simulink model "VDCHyd2020a"  (R2020a)
settings: Solver=daessc  StartTime=0.0  StopTime=simulationEndTime  FixedStep=0.001  RelTol=1e-2
values from neighbouring files (symbols this model uses):
  Bc1_V = [0;0;0;0;0;0]    [initializeSimulationGP.m]
  filtDV = init2ndOrderLowPassFilter(35*2*pi,1,controller.dT)    [initializeLowPassFilters.m]
  filtEnc = init2ndOrderLowPassFilter(35*2*pi,1,controller.dT)    [initializeLowPassFilters.m]
undefined symbols (not defined in the file or in its folder): aux, B11_r_B11Tc1, B11_V, B11_Vr, B11Ftot_r, B12_r_B12Tc2, B12_Rot_Tc2, B12_U_Tc2, B12_V, B12_Vr, B12Ftot_r, B31_r_B31B41, B31_V, B31_Vr, B31FTot_r, B32_r_B32B42, B32_Rot_B42, B32_U_B42, B32_V, B32_Vr, B32FTot_r, B41_r_B41Tc1, B41_V, B41_Vr, B41FTot_r, B42_r_B42Tc2, B42_Rot_Tc2, B42_U_Tc2, B42_V, B42_Vr, B42FTot_r, B52_r_B52P32, B52_Rot_P32, B52_U_P32, B52_V, B52_Vr, B52Ftot_r, Bc1_r_Bc1B11, Bc1_r_Bc1B31, Bc1_Vr, Bc1FTot_r, Bc2_r_Bc2B12, Bc2_r_Bc2B32, Bc2_Rot_B12, Bc2_Rot_B32, Bc2_U_B12, Bc2_U_B32, Bc2_V, Bc2_Vr, Bc2Tot_r, controller, cyl1, cyl2, cylT2, D22_V, D22_Vr, D22Fr, DiscIntNeverNeededParam, dq1, dq11 ... (+125)
libraries: sm_lib x34, nesl_utility x15, simulink x11, dspinverses x1
(part 5 of 12)

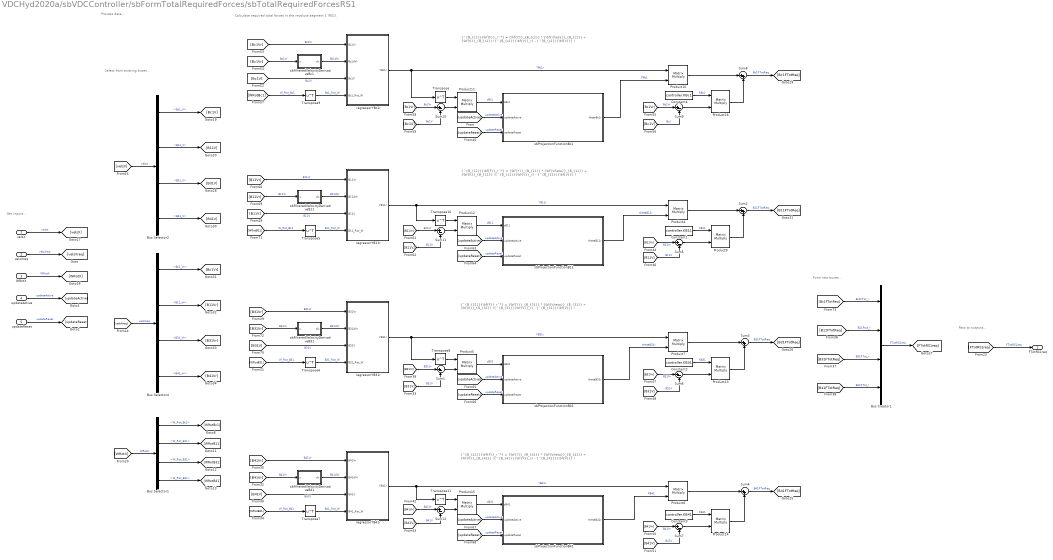
== system VDCHyd2020a/sbVDCController/sbFormTotalRequiredForces/sbTotalRequiredForcesRS1 ==
  note: {^{B_{c1}}{\bf{F}}_r^*} = {\bf{Y}}_{B_{c1}} * {\bf{\theta}}_{B_{c1}} + {\bf{K}}_{B_{c1}} ({^{B_{c1}}{\bf{V}}_r} - {^{B_{c1}}{\bf{V}}} )
  note: Select from existing buses...
  note: Process data...
  note: Get inputs...
  note: Pass to outputs...
  note: Calculate required total forces in the revolute segment 1 (RS1).
  note: Form new buses...
  note: {^{B_{11}}{\bf{F}}_r^*} = {\bf{Y}}_{B_{11}} * {\bf{\theta}}_{B_{11}} + {\bf{K}}_{B_{11}} ({^{B_{11}}{\bf{V}}_r} - {^{B_{11}}{\bf{V}}} )
  note: {^{B_{31}}{\bf{F}}_r^*} = {\bf{Y}}_{B_{31}} * {\bf{\theta}}_{B_{31}} + {\bf{K}}_{B_{31}} ({^{B_{31}}{\bf{V}}_r} - {^{B_{31}}{\bf{V}}} )
  note: {^{B_{41}}{\bf{F}}_r^*} = {\bf{Y}}_{B_{41}} * {\bf{\theta}}_{B_{41}} + {\bf{K}}_{B_{41}} ({^{B_{41}}{\bf{V}}_r} - {^{B_{41}}{\bf{V}}} )
  velsX : Inport
  velsXreq : Inport  Port=2
  WRotX : Inport  Port=3
  updateActive : Inport  Port=4
  updateReset : Inport  Port=5
  Bus Creator1 : BusCreator  Inputs=Bc1FTot_r,B11Ftot_r,B31FTot_r,B41FTot_r
  Bus Selector1 : BusSelector  OutputSignals=WRotXRS1.W_Rot_Bc1,WRotXRS1.W_Rot_B11,WRotXRS1.W_Rot_B31,WRotXRS1.W_Rot_B41
  Bus Selector2 : BusSelector  OutputSignals=velsRS1.Bc1_V,velsRS1.B11_V,velsRS1.B31_V,velsRS1.B41_V
  Bus Selector4 : BusSelector  OutputSignals=velsRS1req.Bc1_Vr,velsRS1req.B11_Vr,velsRS1req.B31_Vr,velsRS1req.B41_Vr
  Constant1 : Constant  Value=controller.KB11
  Constant2 : Constant  Value=controller.KB31
  Constant3 : Constant  Value=controller.KB41
  Constant4 : Constant  Value=controller.KBc1
  Product{4..7,9..16} (12 alike) : Product  Multiplication=Matrix(*)
  Sum{1,5..7,9..12} (8 alike) : Sum  Inputs=|+-
  Sum{2..4,8} (4 alike) : Sum  Inputs=|++
  Transpose{,5..11} (8 alike) : Math  Operator=transpose  SaturateOnIntegerOverflow=on
  regressorYB11r : MATLAB Function  TreatAsAtomicUnit=on
  regressorYB31r : MATLAB Function  TreatAsAtomicUnit=on
  regressorYB41r : MATLAB Function  TreatAsAtomicUnit=on
  regressorYBc1r : MATLAB Function  TreatAsAtomicUnit=on
  sbFilteredVelocityDerivativeB11 : Subsystem
  sbFilteredVelocityDerivativeB31 : Subsystem
  sbFilteredVelocityDerivativeB41 : Subsystem
  sbFilteredVelocityDerivativeBc1 : Subsystem
  sbProjectionFunctionB11 : Subsystem
  sbProjectionFunctionB31 : Subsystem
  sbProjectionFunctionB41 : Subsystem
  sbProjectionFunctionBc1 : Subsystem
  FTotRS1req : Outport
  wires:
  [FTotRS1req] -> FTotRS1req/1  "FTotRS1req"
  velsX/1 -> [velsX]  "velsX"
  [WRotX] -> Bus Selector1/1  "WRotX"
  WRotX/1 -> [WRotX]  "WRotX"
  Bus Selector1/4 -> [WRotB41]  "<W_Rot_B41>"
  Bus Selector1/2 -> [WRotB11]  "<W_Rot_B11>"
  Bus Selector1/1 -> [WRotBc1]  "<W_Rot_Bc1>"
  Bus Selector1/3 -> [WRotB31]  "<W_Rot_B31>"
  regressorYB31r/1(YB31r) -> Transpose8/1, Product7/1  "YB31r"
  [updateReset] -> sbProjectionFunctionB31/3(updateReset)  "updateReset"
  sbFilteredVelocityDerivativeB31/1(du) -> regressorYB31r/2(B31dVr)  "B31dVr"
  [B11V] -> Sum11/2  "B11V"
  [B41V] -> Sum7/2  "B41V"
  [velsX] -> Bus Selector2/1  "velsX"
  [B31V] -> Sum6/2  "B31V"
  Bus Selector4/4 -> [B41Vr]  "<B41_Vr>"
  sbFilteredVelocityDerivativeB41/1(du) -> regressorYB41r/2(B41dVr)  "B41dVr"
  Sum10/1 -> Product11/2
  sbProjectionFunctionB31/1(thetaB31r) -> Product7/2  "thetaB31r"
  Bus Creator1/1 -> [FTotRS1req]  "FTotRS1req"
  Bus Selector4/2 -> [B11Vr]  "<B11_Vr>"
  Bus Selector4/3 -> [B31Vr]  "<B31_Vr>"
  Sum5/1 -> Product9/2
  Sum8/1 -> [Bc1FTotReq]  "Bc1FTotReq"
  [Bc1FTotReq] -> Bus Creator1/1  "Bc1FTot_r"
  [WRotB31] -> Transpose6/1  "W_Rot_B31"
  [B41FTotReq] -> Bus Creator1/4  "B41FTot_r"
  [updateReset] -> sbProjectionFunctionB41/3(updateReset)  "updateReset"
  Bus Selector2/1 -> [Bc1V]  "<Bc1_V>"
  [B31FTotReq] -> Bus Creator1/3  "B31FTot_r"
  Product12/1 -> sbProjectionFunctionB11/1(sB11)  "sB11"
  [WRotBc1] -> Transpose9/1  "W_Rot_Bc1"
  Transpose5/1 -> regressorYB11r/4(B11_Rot_W)  "B11_Rot_W"
  [Bc1Vr] -> Sum9/1  "Bc1Vr"
  [B41Vr] -> regressorYB41r/1(B41Vr)  "B41Vr"
  [B41V] -> Sum12/2  "B41V"
  Transpose/1 -> Product11/1
  [WRotB11] -> Transpose5/1  "W_Rot_B11"
  Bus Selector2/2 -> [B11V]  "<B11_V>"
  [updateReset] -> sbProjectionFunctionBc1/3(updateReset)  "updateReset"
  Bus Selector2/4 -> [B41V]  "<B41_V>"
  [B11Vr] -> regressorYB11r/1(B11Vr)  "B11Vr"
  [Bc1V] -> Sum10/2  "Bc1V"
  Transpose10/1 -> Product12/1
  Sum11/1 -> Product12/2
  [Bc1V] -> regressorYBc1r/3(Bc1V)  "Bc1V"
  regressorYBc1r/1(YBc1r) -> Product10/1, Transpose/1  "YBc1r"
  Product10/1 -> Sum8/1
  Product11/1 -> sbProjectionFunctionBc1/1(sBc1)  "sBc1"
  Transpose8/1 -> Product5/1
  Bus Selector4/1 -> [Bc1Vr]  "<Bc1_Vr>"
  [B11Vr] -> Sum11/1  "B11Vr"
  Product9/1 -> Sum2/2
  Product7/1 -> Sum3/1
  [B31Vr] -> Sum1/1  "B31Vr"
  Sum6/1 -> Product13/2
  [B41Vr] -> Sum7/1  "B41Vr"
  Sum12/1 -> Product15/2
  [updateActive] -> sbProjectionFunctionBc1/2(updateActive)  "updateActive"
  regressorYB11r/1(YB11r) -> Transpose10/1, Product4/1  "YB11r"
  regressorYB41r/1(YB41r) -> Product6/1, Transpose11/1  "YB41r"
  [B41Vr] -> Sum12/1  "B41Vr"
  sbProjectionFunctionBc1/1(thetaBc1r) -> Product10/2  "PBc1"
  Transpose11/1 -> Product15/1
  [WRotB41] -> Transpose7/1  "W_Rot_B41"
  sbFilteredVelocityDerivativeB11/1(du) -> regressorYB11r/2(B11dVr)  "B11dVr"
  [Bc1Vr] -> sbFilteredVelocityDerivativeBc1/1(u)  "Bc1Vr"
  [B41V] -> regressorYB41r/3(B41V)  "B41V"
  Sum7/1 -> Product14/2
  Product15/1 -> sbProjectionFunctionB41/1(sB41)  "sB41"
  [B11Vr] -> Sum5/1  "B11Vr"
  [B31Vr] -> regressorYB31r/1(B31Vr)  "B31Vr"
  [Bc1Vr] -> Sum10/1  "Bc1Vr"
  Constant1/1 -> Product9/1  "KB11"
  [B11V] -> regressorYB11r/3(B11V)  "B11V"
  Transpose7/1 -> regressorYB41r/4(B41_Rot_W)  "B41_Rot_W"
  Transpose9/1 -> regressorYBc1r/4(Bc1_Rot_W)  "Bc1_Rot_W"
  Sum1/1 -> Product5/2
  [B11FTotReq] -> Bus Creator1/2  "B11Ftot_r"
  [B31Vr] -> sbFilteredVelocityDerivativeB31/1(u)  "B31Vr"
  Product6/1 -> Sum4/1
  [B11V] -> Sum5/2  "B11V"
  Product14/1 -> Sum4/2
  [updateActive] -> sbProjectionFunctionB41/2(updateActive)  "updateActive"
  [updateReset] -> sbProjectionFunctionB11/3(updateReset)  "updateReset"
  [velsXreq] -> Bus Selector4/1  "velsXreq"
  Bus Selector2/3 -> [B31V]  "<B31_V>"
  [Bc1Vr] -> regressorYBc1r/1(Bc1Vr)  "Bc1Vr"
  [B31V] -> regressorYB31r/3(B31V)  "B31V"
  sbProjectionFunctionB11/1(thetaB11r) -> Product4/2  "thetaB11r"
  [B41Vr] -> sbFilteredVelocityDerivativeB41/1(u)  "B41Vr"
  Sum9/1 -> Product16/2
  sbFilteredVelocityDerivativeBc1/1(du) -> regressorYBc1r/2(Bc1dVr)  "Bc1dVr"
  Constant4/1 -> Product16/1  "KBc1"
  Constant3/1 -> Product14/1  "KB41"
  Product5/1 -> sbProjectionFunctionB31/1(sB31)  "sB31"
  Sum4/1 -> [B41FTotReq]  "B41FTotReq"
  [B31Vr] -> Sum6/1  "B31Vr"
  [Bc1V] -> Sum9/2  "Bc1"
  Transpose6/1 -> regressorYB31r/4(B31_Rot_W)  "B31_Rot_W"
  [updateActive] -> sbProjectionFunctionB11/2(updateActive)  "updateActive"
  Product16/1 -> Sum8/2
  [B31V] -> Sum1/2  "B31V"
  Product13/1 -> Sum3/2
  Product4/1 -> Sum2/1
  [B11Vr] -> sbFilteredVelocityDerivativeB11/1(u)  "B11Vr"
  Constant2/1 -> Product13/1  "KB31"
  Sum2/1 -> [B11FTotReq]  "B11FTotReq"
  sbProjectionFunctionB41/1(thetaB41r) -> Product6/2  "PB41"
  Sum3/1 -> [B31FTotReq]  "B31FTotReq"
  [updateActive] -> sbProjectionFunctionB31/2(updateActive)  "updateActive"
  velsXreq/1 -> [velsXreq]  "velsXreq"
  updateActive/1 -> [updateActive]  "updateActive"
  updateReset/1 -> [updateReset]  "updateReset"

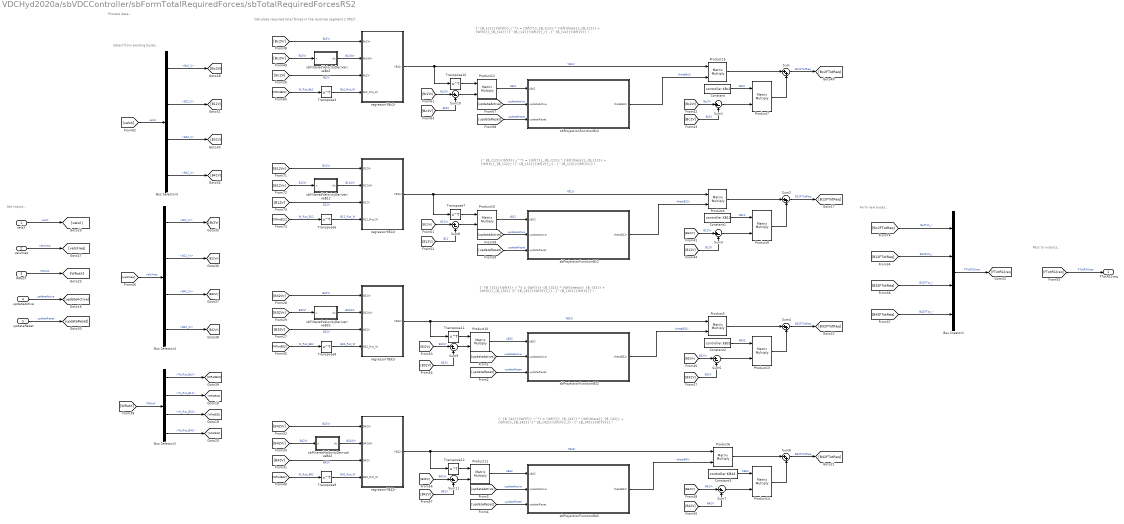
== system VDCHyd2020a/sbVDCController/sbFormTotalRequiredForces/sbTotalRequiredForcesRS2 ==
  note: Form new buses...
  note: Calculate required total forces in the revolute segment 2 (RS2).
  note: Select from existing buses...
  note: Process data...
  note: Pass to outputs...
  note: Get inputs...
  note: {^{B_{c2}}{\bf{F}}_r^*} = {\bf{Y}}_{B_{c2}} * {\bf{\theta}}_{B_{c2}} + {\bf{K}}_{B_{c2}} ({^{B_{c2}}{\bf{V}}_r} - {^{B_{c2}}{\bf{V}}} )
  note: {^{B_{12}}{\bf{F}}_r^*} = {\bf{Y}}_{B_{12}} * {\bf{\theta}}_{B_{12}} + {\bf{K}}_{B_{12}} ({^{B_{12}}{\bf{V}}_r} - {^{B_{12}}{\bf{V}}} )
  note: {^{B_{32}}{\bf{F}}_r^*} = {\bf{Y}}_{B_{32}} * {\bf{\theta}}_{B_{32}} + {\bf{K}}_{B_{32}} ({^{B_{32}}{\bf{V}}_r} - {^{B_{32}}{\bf{V}}} )
  note: {^{B_{42}}{\bf{F}}_r^*} = {\bf{Y}}_{B_{42}} * {\bf{\theta}}_{B_{42}} + {\bf{K}}_{B_{42}} ({^{B_{42}}{\bf{V}}_r} - {^{B_{42}}{\bf{V}}} )
  velsX : Inport
  velsXreq : Inport  Port=2
  WRotX : Inport  Port=3
  updateActive : Inport  Port=4
  updateReset : Inport  Port=5
  Bus Creator1 : BusCreator  Inputs=Bc2Tot_r,B12Ftot_r,B32FTot_r,B42FTot_r
  Bus Selector2 : BusSelector  OutputSignals=WRotXRS1.W_Rot_Bc2,WRotXRS2.W_Rot_B12,WRotXRS2.W_Rot_B32,WRotXRS2.W_Rot_B42
  Bus Selector3 : BusSelector  OutputSignals=velsRS2.Bc2_V,velsRS2.B12_V,velsRS2.B32_V,velsRS2.B42_V
  Bus Selector4 : BusSelector  OutputSignals=velsRS1req.Bc2_Vr,velsRS2req.B12_Vr,velsRS2req.B42_Vr,velsRS2req.B32_Vr
  Constant : Constant  Value=controller.KBc2
  Constant1 : Constant  Value=controller.KB12
  Constant2 : Constant  Value=controller.KB32
  Constant3 : Constant  Value=controller.KB42
  Product{4..7,9..16} (12 alike) : Product  Multiplication=Matrix(*)
  Sum{,2,4,6} (4 alike) : Sum  Inputs=|++
  Sum{1,3,5,7..11} (8 alike) : Sum  Inputs=|+-
  Transpose{3,6..12} (8 alike) : Math  Operator=transpose  SaturateOnIntegerOverflow=on
  regressorYB12r : MATLAB Function  TreatAsAtomicUnit=on
  regressorYB32r : MATLAB Function  TreatAsAtomicUnit=on
  regressorYB42r : MATLAB Function  TreatAsAtomicUnit=on
  regressorYBc2r : MATLAB Function  TreatAsAtomicUnit=on
  sbFilteredVelocityDerivativeB12 : Subsystem
  sbFilteredVelocityDerivativeB32 : Subsystem
  sbFilteredVelocityDerivativeB42 : Subsystem
  sbFilteredVelocityDerivativeBc2 : Subsystem
  sbProjectionFunctionB12 : Subsystem
  sbProjectionFunctionB32 : Subsystem
  sbProjectionFunctionB42 : Subsystem
  sbProjectionFunctionBc2 : Subsystem
  FTotRS2req : Outport
  wires:
  Bus Selector3/1 -> [Bc2V]  "<Bc2_V>"
  Bus Selector2/1 -> [WRotBc2]  "<W_Rot_Bc2>"
  [B42Vr] -> Sum7/1  "B42Vr"
  Product7/1 -> Sum/2
  Bus Creator1/1 -> [FTotRS2req]  "FTotRS2req"
  [B12V] -> regressorYB12r/3(B12V)  "B12V"
  [Bc2V] -> regressorYBc2r/3(Bc2V)  "Bc2V"
  [B32FTotReq] -> Bus Creator1/3  "B32FTot_r"
  [WRotX] -> Bus Selector2/1  "WRotX"
  Transpose10/1 -> Product12/1
  sbProjectionFunctionB12/1(thetaB12r) -> Product4/2  "thetaB12r"
  [Bc2Vr] -> Sum1/1  "Bc2Vr"
  [FTotRS2req] -> FTotRS2req/1  "FTotRS2req"
  [B42FTotReq] -> Bus Creator1/4  "B42FTot_r"
  [Bc2FTotReq] -> Bus Creator1/1  "Bc2Tot_r"
  [B32V] -> Sum9/2  "B32V"
  Sum4/1 -> [B32FTotReq]  "B32FTotReq"
  Bus Selector2/2 -> [WRotB12]  "<W_Rot_B12>"
  [B12Vr] -> Sum3/1  "B12Vr"
  Bus Selector2/4 -> [WRotB42]  "<W_Rot_B42>"
  Transpose6/1 -> regressorYB12r/4(B12_Rot_W)  "B12_Rot_W"
  Sum7/1 -> Product14/2
  [B32Vr] -> sbFilteredVelocityDerivativeB32/1(u)  "B32Vr"
  [WRotB32] -> Transpose8/1  "W_Rot_B32"
  sbFilteredVelocityDerivativeB32/1(du) -> regressorYB32r/2(B32dVr)  "B32dVr"
  [B32Vr] -> regressorYB32r/1(B32Vr)  "B32Vr"
  Product4/1 -> Sum2/1
  [B12Vr] -> Sum8/1  "B12Vr"
  Sum/1 -> [Bc2FTotReq]  "Bc2FTotReq"
  [B42Vr] -> sbFilteredVelocityDerivativeB42/1(u)  "B42Vr"
  [B42Vr] -> regressorYB42r/1(B42Vr)  "B42Vr"
  Constant2/1 -> Product13/1  "KB32"
  Transpose9/1 -> regressorYB42r/4(B42_Rot_W)  "B42_Rot_W"
  [B42V] -> regressorYB42r/3(B42V)  "B42V"
  Constant1/1 -> Product9/1  "KB12"
  [updateReset] -> sbProjectionFunctionB12/3(updateReset)  "updateReset"
  sbProjectionFunctionB32/1(thetaB32r) -> Product5/2  "thetaB32r"
  [updateActive] -> sbProjectionFunctionBc2/2(updateActive)  "updateActive"
  Sum5/1 -> Product13/2
  Sum3/1 -> Product9/2
  Product13/1 -> Sum4/2
  Product11/1 -> sbProjectionFunctionB42/1(sB42)  "sB42"
  Product14/1 -> Sum6/2
  Sum6/1 -> [B42FTotReq]  "B42FTotReq"
  Sum1/1 -> Product7/2
  [B32Vr] -> Sum5/1  "B32Vr"
  Product9/1 -> Sum2/2
  [updateReset] -> sbProjectionFunctionBc2/3(updateReset)  "updateReset"
  Constant3/1 -> Product14/1  "KB42"
  Sum10/1 -> Product12/2
  [Bc2Vr] -> Sum10/1  "Bc2Vr"
  Transpose7/1 -> Product16/1
  [B32Vr] -> Sum9/1  "B32Vr"
  regressorYB32r/1(YB32r) -> Transpose11/1, Product5/1  "YB32r"
  regressorYBc2r/1(YBc2r) -> Product15/1, Transpose10/1  "YBc2r"
  Product16/1 -> sbProjectionFunctionB12/1(sB12)  "sB12"
  [Bc2V] -> Sum10/2  "Bc2V"
  Product5/1 -> Sum4/1
  Transpose11/1 -> Product10/1
  updateReset/1 -> [updateReset]  "updateReset"
  Product12/1 -> sbProjectionFunctionBc2/1(sBc2)  "sBc2"
  [updateActive] -> sbProjectionFunctionB12/2(updateActive)  "updateActive"
  Product10/1 -> sbProjectionFunctionB32/1(sB32)  "sB32"
  [Bc2V] -> Sum1/2  "Bc2V"
  Bus Selector4/4 -> [B42Vr]  "<B32_Vr>"
  [B32V] -> Sum5/2  "B32V"
  sbProjectionFunctionB42/1(thetaB42r) -> Product6/2  "thetaB42r"
  sbProjectionFunctionBc2/1(thetaBc2r) -> Product15/2  "thetaBc2r"
  regressorYB12r/1(YB12r) -> Product4/1, Transpose7/1  "YB12r"
  [velsX] -> Bus Selector3/1  "velsX"
  [WRotB42] -> Transpose9/1  "W_Rot_B42"
  Transpose12/1 -> Product11/1
  regressorYB42r/1(YB42r) -> Product6/1, Transpose12/1  "YB42r"
  Bus Selector3/4 -> [B42V]  "<B42_V>"
  WRotX/1 -> [WRotX]  "WRotX"
  [B12Vr] -> sbFilteredVelocityDerivativeB12/1(u)  "B12Vr"
  Transpose8/1 -> regressorYB32r/4(B32_Rot_W)  "B32_Rot_W"
  Sum9/1 -> Product10/2
  [B42V] -> Sum11/2  "B42V"
  Bus Selector2/3 -> [WRotB32]  "<W_Rot_B32>"
  updateActive/1 -> [updateActive]  "updateActive"
  [WRotBc2] -> Transpose3/1  "W_Rot_Bc2"
  [velsXreq] -> Bus Selector4/1  "velsXreq"
  [B12V] -> Sum8/2  "B12"
  sbFilteredVelocityDerivativeBc2/1(du) -> regressorYBc2r/2(Bc2dVr)  "Bc2dVr"
  Sum8/1 -> Product16/2
  Sum11/1 -> Product11/2
  Sum2/1 -> [B12FTotReq]  "B12FTotReq"
  Bus Selector4/1 -> [Bc2Vr]  "<Bc2_Vr>"
  Constant/1 -> Product7/1  "KBc2"
  [B12V] -> Sum3/2  "B12V"
  [B12Vr] -> regressorYB12r/1(B12Vr)  "B12Vr"
  [Bc2Vr] -> regressorYBc2r/1(Bc2Vr)  "Bc2Vr"
  [B32V] -> regressorYB32r/3(B32V)  "B32V"
  [B42V] -> Sum7/2  "B42V"
  Product6/1 -> Sum6/1
  [WRotB12] -> Transpose6/1  "W_Rot_B12"
  sbFilteredVelocityDerivativeB42/1(du) -> regressorYB42r/2(B42dVr)  "B42dVr"
  sbFilteredVelocityDerivativeB12/1(du) -> regressorYB12r/2(B12dVr)  "B12dVr"
  [B42Vr] -> Sum11/1  "B42Vr"
  Bus Selector3/2 -> [B12V]  "<B12_V>"
  Bus Selector3/3 -> [B32V]  "<B32_V>"
  [Bc2Vr] -> sbFilteredVelocityDerivativeBc2/1(u)  "Bc2Vr"
  Bus Selector4/3 -> [B32Vr]  "<B42_Vr>"
  velsX/1 -> [velsX]  "velsX"
  Transpose3/1 -> regressorYBc2r/4(Bc2_Rot_W)  "Bc2_Rot_W"
  Product15/1 -> Sum/1
  Bus Selector4/2 -> [B12Vr]  "<B12_Vr>"
  velsXreq/1 -> [velsXreq]  "velsXreq"
  [B12FTotReq] -> Bus Creator1/2  "B12Ftot_r"
  [updateReset] -> sbProjectionFunctionB32/3(updateReset)  "updateReset"
  [updateActive] -> sbProjectionFunctionB32/2(updateActive)  "updateActive"
  [updateActive] -> sbProjectionFunctionB42/2(updateActive)  "updateActive"
  [updateReset] -> sbProjectionFunctionB42/3(updateReset)  "updateReset"

== system VDCHyd2020a/sbVDCController/sbFormingControlActions/sbDiscreteDerivativefp1r ==
  fp1r : Inport
  Add : Sum  Inputs=-+
  Gain6 : Gain  Gain=1/(2*controller.dT)
  Integer Delay : Delay  InitialConditionSource=Input port  InitialCondition=0  SampleTime=controller.dT
      settings: InputPortMap=u0,p4
  dfp1r : Outport  PortDimensions=1
  wires:
  Add/1 -> Gain6/1
  fp1r/1 -> Integer Delay/1, Integer Delay/2, Add/2
  Integer Delay/1 -> Add/1
  Gain6/1 -> dfp1r/1

== system VDCHyd2020a/sbVDCController/sbFormingControlActions/sbDiscreteDerivativefp2r ==
  fp2r : Inport
  Add : Sum  Inputs=-+
  Gain6 : Gain  Gain=1/(2*controller.dT)
  Integer Delay : Delay  InitialConditionSource=Input port  InitialCondition=0  SampleTime=controller.dT
      settings: InputPortMap=u0,p4
  dfp2r : Outport  PortDimensions=1
  wires:
  Add/1 -> Gain6/1
  fp2r/1 -> Integer Delay/1, Integer Delay/2, Add/2
  Integer Delay/1 -> Add/1
  Gain6/1 -> dfp2r/1

== system VDCHyd2020a/sbVDCController/sbFormingControlActions/sbDiscreteDerivativefpt2r ==
  fpt2r : Inport
  Add : Sum  Inputs=-+
  Gain6 : Gain  Gain=1/(2*controller.dT)
  Integer Delay : Delay  InitialConditionSource=Input port  InitialCondition=0  SampleTime=controller.dT
      settings: InputPortMap=u0,p4
  dfpt2r : Outport  PortDimensions=1
  wires:
  Gain6/1 -> dfpt2r/1
  Integer Delay/1 -> Add/1
  fpt2r/1 -> Add/2, Integer Delay/2, Integer Delay/1
  Add/1 -> Gain6/1

== system VDCHyd2020a/sbVDCController/sbFormingControlActions/sbFrictionRegressorPS2 ==
  note: (40) in Zhu, Piedboeuf (2005)
  note: (4) in Zhu, Piedboeuf (2005)
  note: (71) and (72) in Zhu, Piedboeuf (2005)
  dxt2 : Inport
  fpt2 : Inport  Port=2
  frictionRegressorFunctionPS2 : MATLAB Function  TreatAsAtomicUnit=on
  sbAverageDeformationOfBristlesPS2 : Subsystem
  sbFrictionSwitchingFunctionPS2 : Subsystem
  Yft2 : Outport
  wires:
  dxt2/1 -> [dxt2]  "dxt2"
  [dxt2] -> sbAverageDeformationOfBristlesPS2/1(dxt2)  "dxt2"
  sbAverageDeformationOfBristlesPS2/1(zt2) -> [zt2]  "zt2"
  [dxt2] -> sbFrictionSwitchingFunctionPS2/1(dxt2)  "dxt2"
  sbFrictionSwitchingFunctionPS2/1(LPS2) -> [LPS2]  "LPS2"
  [dxt2] -> frictionRegressorFunctionPS2/1(v)  "dxt2"
  [zt2] -> frictionRegressorFunctionPS2/2(z)  "zt2"
  [LPS2] -> frictionRegressorFunctionPS2/3(L)  "LPS2"
  fpt2/1 -> [fpt2]  "fpt2"
  [fpt2] -> frictionRegressorFunctionPS2/4(Fd)  "fpt2"
  frictionRegressorFunctionPS2/1(Yf) -> [Yft2]  "Yft2"
  [Yft2] -> Yft2/1  "Yft2"

== system VDCHyd2020a/sbVDCController/sbFormingControlActions/sbFrictionRegressorRS1 ==
  note: (40) in Zhu, Piedboeuf (2005)
  note: (4) in Zhu, Piedboeuf (2005)
  note: (71) and (72) in Zhu, Piedboeuf (2005)
  dx1 : Inport
  fp1 : Inport  Port=2
  frictionRegressorFunctionRS1 : MATLAB Function  TreatAsAtomicUnit=on
  sbAverageDeformationOfBristlesRS2 : Subsystem
  sbFrictionSwitchingFunctionRS2 : Subsystem
  Yf1 : Outport
  wires:
  dx1/1 -> [dx1]  "dx1"
  [dx1] -> sbAverageDeformationOfBristlesRS2/1(dx1)  "dx1"
  sbAverageDeformationOfBristlesRS2/1(z1) -> [z1]  "z1"
  [dx1] -> sbFrictionSwitchingFunctionRS2/1(dx1)  "dx1"
  sbFrictionSwitchingFunctionRS2/1(LRS1) -> [LRS1]  "LRS1"
  [dx1] -> frictionRegressorFunctionRS1/1(v)  "dx1"
  [z1] -> frictionRegressorFunctionRS1/2(z)  "z1"
  [LRS1] -> frictionRegressorFunctionRS1/3(L)  "LRS1"
  fp1/1 -> [fp1]  "fp1"
  [fp1] -> frictionRegressorFunctionRS1/4(Fd)  "fp1"
  frictionRegressorFunctionRS1/1(Yf) -> [Yf1]  "Yf1"
  [Yf1] -> Yf1/1  "Yf1"

== system VDCHyd2020a/sbVDCController/sbFormingControlActions/sbFrictionRegressorRS2 ==
  note: (40) in Zhu, Piedboeuf (2005)
  note: (4) in Zhu, Piedboeuf (2005)
  note: (71) and (72) in Zhu, Piedboeuf (2005)
  dx2 : Inport
  fp2 : Inport  Port=2
  frictionRegressorFunctionRS2 : MATLAB Function  TreatAsAtomicUnit=on
  sbAverageDeformationOfBristlesRS2 : Subsystem
  sbFrictionSwitchingFunctionRS2 : Subsystem
  Yf2 : Outport
  wires:
  dx2/1 -> [dx2]  "dx2"
  [dx2] -> sbAverageDeformationOfBristlesRS2/1(dx2)  "dx2"
  sbAverageDeformationOfBristlesRS2/1(z2) -> [z2]  "z2"
  [dx2] -> sbFrictionSwitchingFunctionRS2/1(dx2)  "dx2"
  sbFrictionSwitchingFunctionRS2/1(LRS2) -> [LRS2]  "LRS2"
  [dx2] -> frictionRegressorFunctionRS2/1(v)  "dx2"
  [z2] -> frictionRegressorFunctionRS2/2(z)  "z2"
  [LRS2] -> frictionRegressorFunctionRS2/3(L)  "LRS2"
  fp2/1 -> [fp2]  "fp2"
  [fp2] -> frictionRegressorFunctionRS2/4(Fd)  "fp2"
  frictionRegressorFunctionRS2/1(Yf) -> [Yf2]  "Yf2"
  [Yf2] -> Yf2/1  "Yf2"

== system VDCHyd2020a/sbVDCController/sbFormingControlActions/sbLowPassFilter2 ==
  dfp2r : Inport
  Delay : Delay  InitialConditionSource=Input port  SampleTime=filtDF.dT
      settings: InputPortMap=u0,p4
  Delay1 : Delay  DelayLength=1  InitialConditionSource=Input port  SampleTime=filtDF.dT
      settings: InputPortMap=u0,p4
  Delay2 : Delay  DelayLength=0  InitialConditionSource=Input port  SampleTime=filtDF.dT
      settings: InputPortMap=u0,p4
  Delay3 : Delay  InitialConditionSource=Input port  SampleTime=filtDF.dT
      settings: InputPortMap=u0,p4
  Delay4 : Delay  DelayLength=1  InitialConditionSource=Input port  SampleTime=filtDF.dT
      settings: InputPortMap=u0,p4
  Gain : Gain  Gain=filtDF.a0
  Gain1 : Gain  Gain=filtDF.b1
  Gain2 : Gain  Gain=filtDF.b2
  Gain3 : Gain  Gain=filtDF.b0
  Gain4 : Gain  Gain=filtDF.a1
  Sum : Sum  Inputs=|--+++
  dfp2rFilt : Outport
  wires:
  Delay2/1 -> Gain2/1
  Delay3/1 -> Gain3/1
  Gain1/1 -> Sum/4
  Delay/1 -> Gain/1
  Gain2/1 -> Sum/3
  Gain3/1 -> Sum/5
  Sum/1 -> dfp2rFilt/1, Delay4/1, Delay/1  "df2pFilt"
  Gain4/1 -> Sum/1
  Delay1/1 -> Gain1/1
  Delay4/1 -> Gain4/1
  Gain/1 -> Sum/2
  dfp2r/1 -> Delay4/2, Delay/2, Delay2/1, Delay2/2, Delay1/1, Delay3/2, Delay3/1, Delay1/2  "df2p"

== system VDCHyd2020a/sbVDCController/sbFormingControlActions/sbLowPassFilterdfp1r ==
  dfp1r : Inport
  Delay : Delay  InitialConditionSource=Input port  SampleTime=filtDF.dT
      settings: InputPortMap=u0,p4
  Delay1 : Delay  DelayLength=1  InitialConditionSource=Input port  SampleTime=filtDF.dT
      settings: InputPortMap=u0,p4
  Delay2 : Delay  DelayLength=0  InitialConditionSource=Input port  SampleTime=filtDF.dT
      settings: InputPortMap=u0,p4
  Delay3 : Delay  InitialConditionSource=Input port  SampleTime=filtDF.dT
      settings: InputPortMap=u0,p4
  Delay4 : Delay  DelayLength=1  InitialConditionSource=Input port  SampleTime=filtDF.dT
      settings: InputPortMap=u0,p4
  Gain : Gain  Gain=filtDF.a0
  Gain1 : Gain  Gain=filtDF.b1
  Gain2 : Gain  Gain=filtDF.b2
  Gain3 : Gain  Gain=filtDF.b0
  Gain4 : Gain  Gain=filtDF.a1
  Sum : Sum  Inputs=|--+++
  dfp1rFilt : Outport
  wires:
  dfp1r/1 -> Delay1/2, Delay3/1, Delay3/2, Delay1/1, Delay2/2, Delay2/1, Delay/2, Delay4/2  "df1p"
  Gain/1 -> Sum/2
  Delay4/1 -> Gain4/1
  Delay1/1 -> Gain1/1
  Gain4/1 -> Sum/1
  Sum/1 -> Delay/1, Delay4/1, dfp1rFilt/1  "df1pFilt"
  Gain3/1 -> Sum/5
  Gain2/1 -> Sum/3
  Delay/1 -> Gain/1
  Gain1/1 -> Sum/4
  Delay3/1 -> Gain3/1
  Delay2/1 -> Gain2/1

== system VDCHyd2020a/sbVDCController/sbFormingControlActions/sbLowPassFilterdfpt2r ==
  dfpt2r : Inport
  Delay : Delay  InitialConditionSource=Input port  SampleTime=filtDF.dT
      settings: InputPortMap=u0,p4
  Delay1 : Delay  DelayLength=1  InitialConditionSource=Input port  SampleTime=filtDF.dT
      settings: InputPortMap=u0,p4
  Delay2 : Delay  DelayLength=0  InitialConditionSource=Input port  SampleTime=filtDF.dT
      settings: InputPortMap=u0,p4
  Delay3 : Delay  InitialConditionSource=Input port  SampleTime=filtDF.dT
      settings: InputPortMap=u0,p4
  Delay4 : Delay  DelayLength=1  InitialConditionSource=Input port  SampleTime=filtDF.dT
      settings: InputPortMap=u0,p4
  Gain : Gain  Gain=filtDF.a0
  Gain1 : Gain  Gain=filtDF.b1
  Gain2 : Gain  Gain=filtDF.b2
  Gain3 : Gain  Gain=filtDF.b0
  Gain4 : Gain  Gain=filtDF.a1
  Sum : Sum  Inputs=|--+++
  dfpt2rFilt : Outport
  wires:
  dfpt2r/1 -> Delay1/2, Delay3/1, Delay3/2, Delay1/1, Delay2/2, Delay2/1, Delay/2, Delay4/2  "dft2p"
  Gain/1 -> Sum/2
  Delay4/1 -> Gain4/1
  Delay1/1 -> Gain1/1
  Gain4/1 -> Sum/1
  Sum/1 -> Delay/1, Delay4/1, dfpt2rFilt/1  "dft2pFilt"
  Gain3/1 -> Sum/5
  Gain2/1 -> Sum/3
  Delay/1 -> Gain/1
  Gain1/1 -> Sum/4
  Delay3/1 -> Gain3/1
  Delay2/1 -> Gain2/1

== system VDCHyd2020a/sbVDCController/sbFormingControlActions/sbProjectionFunctiond1 ==
  sd1 : Inport  PortDimensions=4
  updateActive : Inport  Port=2
  updateReset : Inport  Port=3
  Constant1 : Constant  Value=update.thetad1Nominal
  Switch1 : Switch  Criteria=u2 > Threshold
  discreteIntegratorPd1 : DiscreteIntegrator  IntegratorMethod=Integration: Trapezoidal  gainval=update.rhod1  ExternalReset=level  InitialConditionSource=external  InitialCondition=update.thetad1Nominal  SampleTime=controller.dT  LimitOutput=on  UpperSaturationLimit=update.thetad1UpperBound  LowerSaturationLimit=update.thetad1LowerBound  ICPrevOutput=DiscIntNeverNeededParam  ICPrevScaledInput=DiscIntNeverNeededParam
  thetad1 : Outport
  wires:
  sd1/1 -> discreteIntegratorPd1/1  "sd1"
  updateReset/1 -> discreteIntegratorPd1/2  "updateReset"
  discreteIntegratorPd1/1 -> Switch1/1  "thetad1Updated"
  Switch1/1 -> thetad1/1  "thetad1"
  updateActive/1 -> Switch1/2  "updateActive"
  Constant1/1 -> discreteIntegratorPd1/3, Switch1/3  "thetad1Nominal"

== system VDCHyd2020a/sbVDCController/sbFormingControlActions/sbProjectionFunctiond2 ==
  sd2 : Inport  PortDimensions=4
  updateActive : Inport  Port=2
  updateReset : Inport  Port=3
  Constant1 : Constant  Value=update.thetad2Nominal
  Switch1 : Switch  Criteria=u2 > Threshold
  discreteIntegratorPd2 : DiscreteIntegrator  IntegratorMethod=Integration: Trapezoidal  gainval=update.rhod2  ExternalReset=level  InitialConditionSource=external  InitialCondition=update.thetad2Nominal  SampleTime=controller.dT  LimitOutput=on  UpperSaturationLimit=update.thetad2UpperBound  LowerSaturationLimit=update.thetad2LowerBound  ICPrevOutput=DiscIntNeverNeededParam  ICPrevScaledInput=DiscIntNeverNeededParam
  thetad2 : Outport
  wires:
  Constant1/1 -> Switch1/3, discreteIntegratorPd2/3  "thetad2Nominal"
  updateActive/1 -> Switch1/2  "updateActive"
  Switch1/1 -> thetad2/1  "thetad2"
  discreteIntegratorPd2/1 -> Switch1/1  "thetad2Updated"
  updateReset/1 -> discreteIntegratorPd2/2  "updateReset"
  sd2/1 -> discreteIntegratorPd2/1  "sd2"

== system VDCHyd2020a/sbVDCController/sbFormingControlActions/sbProjectionFunctiondt2 ==
  sdt2 : Inport  PortDimensions=4
  updateActive : Inport  Port=2
  updateReset : Inport  Port=3
  Constant1 : Constant  Value=update.thetadT2Nominal
  Discrete-Time Integrator : DiscreteIntegrator  IntegratorMethod=Integration: Trapezoidal  gainval=update.rhodT2  ExternalReset=level  InitialConditionSource=external  InitialCondition=update.thetadT2Nominal  SampleTime=controller.dT  LimitOutput=on  UpperSaturationLimit=update.thetadT2UpperBound  LowerSaturationLimit=update.thetadT2LowerBound  ICPrevOutput=DiscIntNeverNeededParam  ICPrevScaledInput=DiscIntNeverNeededParam
  Switch1 : Switch  Criteria=u2 > Threshold
  thetadT2 : Outport
  wires:
  sdt2/1 -> Discrete-Time Integrator/1  "sdt2"
  updateReset/1 -> Discrete-Time Integrator/2  "updateReset"
  Discrete-Time Integrator/1 -> Switch1/1  "thetadT2Updated"
  Switch1/1 -> thetadT2/1  "thetadT2"
  updateActive/1 -> Switch1/2  "updateActive"
  Constant1/1 -> Switch1/3, Discrete-Time Integrator/3  "thetadT2Nominal"

== system VDCHyd2020a/sbVDCController/sbFormingControlActions/sbProjectionFunctionfRS1 ==
  sf1 : Inport
  updateActive : Inport  Port=2
  updateReset : Inport  Port=3
  Constant1 : Constant  Value=update.thetaf1Nominal
  Switch1 : Switch  Criteria=u2 > Threshold
  discreteIntegratorPf1 : DiscreteIntegrator  IntegratorMethod=Integration: Trapezoidal  gainval=update.rhof1  ExternalReset=level  InitialConditionSource=external  InitialCondition=update.thetaf1Nominal  SampleTime=controller.dT  LimitOutput=on  UpperSaturationLimit=update.thetaf1UpperBound  LowerSaturationLimit=update.thetaf1LowerBound  ICPrevOutput=DiscIntNeverNeededParam  ICPrevScaledInput=DiscIntNeverNeededParam
  thetaf1 : Outport
  wires:
  sf1/1 -> discreteIntegratorPf1/1  "sf1"
  updateReset/1 -> discreteIntegratorPf1/2  "updateReset"
  discreteIntegratorPf1/1 -> Switch1/1  "thetaf1Updated"
  Switch1/1 -> thetaf1/1  "thetaf1"
  updateActive/1 -> Switch1/2  "updateActive"
  Constant1/1 -> discreteIntegratorPf1/3, Switch1/3  "thetaf1Nominal"

== system VDCHyd2020a/sbVDCController/sbFormingControlActions/sbProjectionFunctionfRS2 ==
  sf2 : Inport
  updateActive : Inport  Port=2
  updateReset : Inport  Port=3
  Constant1 : Constant  Value=update.thetaf2Nominal
  Switch1 : Switch  Criteria=u2 > Threshold
  discreteIntegratorPf2 : DiscreteIntegrator  IntegratorMethod=Integration: Trapezoidal  gainval=update.rhof2  ExternalReset=level  InitialConditionSource=external  InitialCondition=update.thetaf2Nominal  SampleTime=controller.dT  LimitOutput=on  UpperSaturationLimit=update.thetaf2UpperBound  LowerSaturationLimit=update.thetaf2LowerBound  ICPrevOutput=DiscIntNeverNeededParam  ICPrevScaledInput=DiscIntNeverNeededParam
  thetaf2 : Outport
  wires:
  Constant1/1 -> Switch1/3, discreteIntegratorPf2/3  "thetaf2Nominal"
  updateActive/1 -> Switch1/2  "updateActive"
  Switch1/1 -> thetaf2/1  "thetaf2"
  discreteIntegratorPf2/1 -> Switch1/1  "thetaf2Updated"
  updateReset/1 -> discreteIntegratorPf2/2  "updateReset"
  sf2/1 -> discreteIntegratorPf2/1  "sf2"

== system VDCHyd2020a/sbVDCController/sbFormingControlActions/sbProjectionFunctionfRS3 ==
  sfT2 : Inport
  updateActive : Inport  Port=2
  updateReset : Inport  Port=3
  Constant1 : Constant  Value=update.thetafT2Nominal
  Switch1 : Switch  Criteria=u2 > Threshold
  discreteIntegratorPfT2 : DiscreteIntegrator  IntegratorMethod=Integration: Trapezoidal  gainval=update.rhofT2  ExternalReset=level  InitialConditionSource=external  InitialCondition=update.thetafT2Nominal  SampleTime=controller.dT  LimitOutput=on  UpperSaturationLimit=update.thetafT2UpperBound  LowerSaturationLimit=update.thetafT2LowerBound  ICPrevOutput=DiscIntNeverNeededParam  ICPrevScaledInput=DiscIntNeverNeededParam
  thetafT2 : Outport
  wires:
  sfT2/1 -> discreteIntegratorPfT2/1  "sfT2"
  updateReset/1 -> discreteIntegratorPfT2/2  "updateReset"
  discreteIntegratorPfT2/1 -> Switch1/1  "thetaf2Updated"
  Switch1/1 -> thetafT2/1  "thetafT2"
  updateActive/1 -> Switch1/2  "updateActive"
  Constant1/1 -> discreteIntegratorPfT2/3, Switch1/3  "thetafT2Nominal"

== system VDCHyd2020a/sbVDCController/sbFormingControlActions/sbProjectionFunctionv1 ==
  sv1 : Inport  PortDimensions=4
  updateActive : Inport  Port=2
  updateReset : Inport  Port=3
  Constant1 : Constant  Value=update.thetav1Nominal
  Switch1 : Switch  Criteria=u2 > Threshold
  Unit Delay : UnitDelay  InitialCondition=update.thetav1Nominal  SampleTime=controller.dT  HasFrameUpgradeWarning=on
  discreteIntegratorPv1 : DiscreteIntegrator  IntegratorMethod=Integration: Trapezoidal  gainval=update.rhov1  ExternalReset=level  InitialConditionSource=external  InitialCondition=update.thetav1Nominal  SampleTime=controller.dT  LimitOutput=on  UpperSaturationLimit=update.thetav1UpperBound  LowerSaturationLimit=update.thetav1LowerBound  ICPrevOutput=DiscIntNeverNeededParam  ICPrevScaledInput=DiscIntNeverNeededParam
  thetav1 : Outport
  wires:
  Constant1/1 -> discreteIntegratorPv1/3, Switch1/3  "thetav1Nominal"
  updateActive/1 -> Switch1/2  "updateActive"
  Switch1/1 -> thetav1/1  "thetav1"
  discreteIntegratorPv1/1 -> Unit Delay/1
  updateReset/1 -> discreteIntegratorPv1/2  "updateReset"
  sv1/1 -> discreteIntegratorPv1/1  "sv1"
  Unit Delay/1 -> Switch1/1  "thetav1Update"

== system VDCHyd2020a/sbVDCController/sbFormingControlActions/sbProjectionFunctionv2 ==
  sv2 : Inport  PortDimensions=4
  updateActive : Inport  Port=2
  updateReset : Inport  Port=3
  Constant1 : Constant  Value=update.thetav2Nominal
  Discrete-Time Integrator : DiscreteIntegrator  IntegratorMethod=Integration: Trapezoidal  gainval=update.rhov2  ExternalReset=level  InitialConditionSource=external  InitialCondition=update.thetav2Nominal  SampleTime=controller.dT  LimitOutput=on  UpperSaturationLimit=update.thetav2UpperBound  LowerSaturationLimit=update.thetav2LowerBound  ICPrevOutput=DiscIntNeverNeededParam  ICPrevScaledInput=DiscIntNeverNeededParam
  Switch1 : Switch  Criteria=u2 > Threshold
  Unit Delay : UnitDelay  InitialCondition=update.thetav2Nominal  SampleTime=controller.dT  HasFrameUpgradeWarning=on
  thetav2 : Outport
  wires:
  Constant1/1 -> Switch1/3, Discrete-Time Integrator/3  "thetav2Nominal"
  updateActive/1 -> Switch1/2  "updateActive"
  Switch1/1 -> thetav2/1  "thetav2"
  Discrete-Time Integrator/1 -> Unit Delay/1
  updateReset/1 -> Discrete-Time Integrator/2  "updateReset"
  sv2/1 -> Discrete-Time Integrator/1  "sv2"
  Unit Delay/1 -> Switch1/1  "thetav2Updated"

== system VDCHyd2020a/sbVDCController/sbFormingControlActions/sbProjectionFunctionvt2 ==
  svt2 : Inport  PortDimensions=4
  updateActive : Inport  Port=2
  updateReset : Inport  Port=3
  Constant1 : Constant  Value=update.thetavT2Nominal
  Discrete-Time Integrator : DiscreteIntegrator  IntegratorMethod=Integration: Trapezoidal  gainval=update.rhovT2  ExternalReset=level  InitialConditionSource=external  InitialCondition=update.thetavT2Nominal  SampleTime=controller.dT  LimitOutput=on  UpperSaturationLimit=update.thetavT2UpperBound  LowerSaturationLimit=update.thetavT2LowerBound  ICPrevOutput=DiscIntNeverNeededParam  ICPrevScaledInput=DiscIntNeverNeededParam
  Switch1 : Switch  Criteria=u2 > Threshold
  Unit Delay : UnitDelay  InitialCondition=update.thetavT2Nominal  SampleTime=controller.dT  HasFrameUpgradeWarning=on
  thetavt2 : Outport
  wires:
  svt2/1 -> Discrete-Time Integrator/1
  Switch1/1 -> thetavt2/1  "thetavT2"
  Unit Delay/1 -> Switch1/1  "thetavT2Updated"
  updateActive/1 -> Switch1/2
  Constant1/1 -> Switch1/3, Discrete-Time Integrator/3  "thetavT2Nominal"
  updateReset/1 -> Discrete-Time Integrator/2
  Discrete-Time Integrator/1 -> Unit Delay/1

== system VDCHyd2020a/sbVDCController/sbFormingControlActions/sbpRLowPassFilter ==
  pRMeas : Inport
  Delay : Delay  InitialConditionSource=Input port  SampleTime=filtPres.dT
      settings: InputPortMap=u0,p4
  Delay1 : Delay  DelayLength=1  InitialConditionSource=Input port  SampleTime=filtPres.dT
      settings: InputPortMap=u0,p4
  Delay2 : Delay  DelayLength=0  InitialConditionSource=Input port  SampleTime=filtPres.dT
      settings: InputPortMap=u0,p4
  Delay3 : Delay  InitialConditionSource=Input port  SampleTime=filtPres.dT
      settings: InputPortMap=u0,p4
  Delay4 : Delay  DelayLength=1  InitialConditionSource=Input port  SampleTime=filtPres.dT
      settings: InputPortMap=u0,p4
  Gain : Gain  Gain=filtPres.a0
  Gain1 : Gain  Gain=filtPres.b1
  Gain2 : Gain  Gain=filtPres.b2
  Gain3 : Gain  Gain=filtPres.b0
  Gain4 : Gain  Gain=filtPres.a1
  Sum : Sum  Inputs=|--+++
  pRFilt : Outport
  wires:
  Gain3/1 -> Sum/5
  Sum/1 -> Delay/1, Delay4/1, pRFilt/1  "pRFilt"
  Gain2/1 -> Sum/3
  Delay/1 -> Gain/1
  Gain1/1 -> Sum/4
  Gain/1 -> Sum/2
  Delay1/1 -> Gain1/1
  Delay4/1 -> Gain4/1
  Delay2/1 -> Gain2/1
  Gain4/1 -> Sum/1
  Delay3/1 -> Gain3/1
  pRMeas/1 -> Delay1/2, Delay3/1, Delay3/2, Delay1/1, Delay2/2, Delay2/1, Delay/2, Delay4/2  "pRMeas"

== system VDCHyd2020a/sbVDCController/sbFormingControlActions/sbpSLowPassFilter ==
  pSMeas : Inport
  Delay : Delay  InitialConditionSource=Input port  SampleTime=filtPres.dT
      settings: InputPortMap=u0,p4
  Delay1 : Delay  DelayLength=1  InitialConditionSource=Input port  SampleTime=filtPres.dT
      settings: InputPortMap=u0,p4
  Delay2 : Delay  DelayLength=0  InitialConditionSource=Input port  SampleTime=filtPres.dT
      settings: InputPortMap=u0,p4
  Delay3 : Delay  InitialConditionSource=Input port  SampleTime=filtPres.dT
      settings: InputPortMap=u0,p4
  Delay4 : Delay  DelayLength=1  InitialConditionSource=Input port  SampleTime=filtPres.dT
      settings: InputPortMap=u0,p4
  Gain : Gain  Gain=filtPres.a0
  Gain1 : Gain  Gain=filtPres.b1
  Gain2 : Gain  Gain=filtPres.b2
  Gain3 : Gain  Gain=filtPres.b0
  Gain4 : Gain  Gain=filtPres.a1
  Sum : Sum  Inputs=|--+++
  pSFilt : Outport
  wires:
  pSMeas/1 -> Delay4/2, Delay/2, Delay2/1, Delay2/2, Delay1/1, Delay3/2, Delay3/1, Delay1/2  "pSMeas"
  Delay3/1 -> Gain3/1
  Gain4/1 -> Sum/1
  Delay2/1 -> Gain2/1
  Delay4/1 -> Gain4/1
  Delay1/1 -> Gain1/1
  Gain/1 -> Sum/2
  Gain1/1 -> Sum/4
  Delay/1 -> Gain/1
  Gain2/1 -> Sum/3
  Sum/1 -> pSFilt/1, Delay4/1, Delay/1  "pSFilt"
  Gain3/1 -> Sum/5

== system VDCHyd2020a/sbVDCController/sbFormingControlActions/sbpa1LowPassFilter ==
  pa1Meas : Inport
  Delay : Delay  InitialConditionSource=Input port  SampleTime=filtPres.dT
      settings: InputPortMap=u0,p4
  Delay1 : Delay  DelayLength=1  InitialConditionSource=Input port  SampleTime=filtPres.dT
      settings: InputPortMap=u0,p4
  Delay2 : Delay  DelayLength=0  InitialConditionSource=Input port  SampleTime=filtPres.dT
      settings: InputPortMap=u0,p4
  Delay3 : Delay  InitialConditionSource=Input port  SampleTime=filtPres.dT
      settings: InputPortMap=u0,p4
  Delay4 : Delay  DelayLength=1  InitialConditionSource=Input port  SampleTime=filtPres.dT
      settings: InputPortMap=u0,p4
  Gain : Gain  Gain=filtPres.a0
  Gain1 : Gain  Gain=filtPres.b1
  Gain2 : Gain  Gain=filtPres.b2
  Gain3 : Gain  Gain=filtPres.b0
  Gain4 : Gain  Gain=filtPres.a1
  Sum : Sum  Inputs=|--+++
  pa1Filt : Outport
  wires:
  Gain2/1 -> Sum/3
  Delay3/1 -> Gain3/1
  Gain1/1 -> Sum/4
  pa1Meas/1 -> Delay4/2, Delay/2, Delay2/1, Delay2/2, Delay1/1, Delay3/2, Delay3/1, Delay1/2  "pa1Meas"
  Gain/1 -> Sum/2
  Sum/1 -> pa1Filt/1, Delay4/1, Delay/1  "pa1Filt"
  Gain3/1 -> Sum/5
  Gain4/1 -> Sum/1
  Delay2/1 -> Gain2/1
  Delay1/1 -> Gain1/1
  Delay/1 -> Gain/1
  Delay4/1 -> Gain4/1

== system VDCHyd2020a/sbVDCController/sbFormingControlActions/sbpa2LowPassFilter ==
  pa2Meas : Inport
  Delay : Delay  InitialConditionSource=Input port  SampleTime=filtPres.dT
      settings: InputPortMap=u0,p4
  Delay1 : Delay  DelayLength=1  InitialConditionSource=Input port  SampleTime=filtPres.dT
      settings: InputPortMap=u0,p4
  Delay2 : Delay  DelayLength=0  InitialConditionSource=Input port  SampleTime=filtPres.dT
      settings: InputPortMap=u0,p4
  Delay3 : Delay  InitialConditionSource=Input port  SampleTime=filtPres.dT
      settings: InputPortMap=u0,p4
  Delay4 : Delay  DelayLength=1  InitialConditionSource=Input port  SampleTime=filtPres.dT
      settings: InputPortMap=u0,p4
  Gain : Gain  Gain=filtPres.a0
  Gain1 : Gain  Gain=filtPres.b1
  Gain2 : Gain  Gain=filtPres.b2
  Gain3 : Gain  Gain=filtPres.b0
  Gain4 : Gain  Gain=filtPres.a1
  Sum : Sum  Inputs=|--+++
  pa2Filt : Outport
  wires:
  Gain1/1 -> Sum/4
  Delay3/1 -> Gain3/1
  Delay/1 -> Gain/1
  Gain/1 -> Sum/2
  Delay2/1 -> Gain2/1
  Delay1/1 -> Gain1/1
  Gain4/1 -> Sum/1
  Delay4/1 -> Gain4/1
  Sum/1 -> pa2Filt/1, Delay4/1, Delay/1  "pa2_filt"
  Gain3/1 -> Sum/5
  Gain2/1 -> Sum/3
  pa2Meas/1 -> Delay4/2, Delay/2, Delay2/1, Delay2/2, Delay1/1, Delay3/2, Delay3/1, Delay1/2  "pa2_meas"

== system VDCHyd2020a/sbVDCController/sbFormingControlActions/sbpat2LowPassFilter ==
  pat2Meas : Inport
  Delay : Delay  InitialConditionSource=Input port  SampleTime=filtPres.dT
      settings: InputPortMap=u0,p4
  Delay1 : Delay  DelayLength=1  InitialConditionSource=Input port  SampleTime=filtPres.dT
      settings: InputPortMap=u0,p4
  Delay2 : Delay  DelayLength=0  InitialConditionSource=Input port  SampleTime=filtPres.dT
      settings: InputPortMap=u0,p4
  Delay3 : Delay  InitialConditionSource=Input port  SampleTime=filtPres.dT
      settings: InputPortMap=u0,p4
  Delay4 : Delay  DelayLength=1  InitialConditionSource=Input port  SampleTime=filtPres.dT
      settings: InputPortMap=u0,p4
  Gain : Gain  Gain=filtPres.a0
  Gain1 : Gain  Gain=filtPres.b1
  Gain2 : Gain  Gain=filtPres.b2
  Gain3 : Gain  Gain=filtPres.b0
  Gain4 : Gain  Gain=filtPres.a1
  Sum : Sum  Inputs=|--+++
  pat2Filt : Outport
  wires:
  pat2Meas/1 -> Delay4/2, Delay/2, Delay2/1, Delay2/2, Delay1/1, Delay3/2, Delay3/1, Delay1/2  "paT2_meas"
  Delay3/1 -> Gain3/1
  Gain2/1 -> Sum/3
  Gain/1 -> Sum/2
  Delay4/1 -> Gain4/1
  Gain4/1 -> Sum/1
  Delay2/1 -> Gain2/1
  Gain3/1 -> Sum/5
  Gain1/1 -> Sum/4
  Sum/1 -> pat2Filt/1, Delay4/1, Delay/1  "paT2_filt"
  Delay1/1 -> Gain1/1
  Delay/1 -> Gain/1

== system VDCHyd2020a/sbVDCController/sbFormingControlActions/sbpb1LowPassFilter ==
  pb1Meas : Inport
  Delay : Delay  InitialConditionSource=Input port  SampleTime=filtPres.dT
      settings: InputPortMap=u0,p4
  Delay1 : Delay  DelayLength=1  InitialConditionSource=Input port  SampleTime=filtPres.dT
      settings: InputPortMap=u0,p4
  Delay2 : Delay  DelayLength=0  InitialConditionSource=Input port  SampleTime=filtPres.dT
      settings: InputPortMap=u0,p4
  Delay3 : Delay  InitialConditionSource=Input port  SampleTime=filtPres.dT
      settings: InputPortMap=u0,p4
  Delay4 : Delay  DelayLength=1  InitialConditionSource=Input port  SampleTime=filtPres.dT
      settings: InputPortMap=u0,p4
  Gain : Gain  Gain=filtPres.a0
  Gain1 : Gain  Gain=filtPres.b1
  Gain2 : Gain  Gain=filtPres.b2
  Gain3 : Gain  Gain=filtPres.b0
  Gain4 : Gain  Gain=filtPres.a1
  Sum : Sum  Inputs=|--+++
  pb1Filt : Outport
  wires:
  Delay3/1 -> Gain3/1
  Delay1/1 -> Gain1/1
  Delay2/1 -> Gain2/1
  Delay4/1 -> Gain4/1
  Gain4/1 -> Sum/1
  Gain3/1 -> Sum/5
  Gain/1 -> Sum/2
  Gain2/1 -> Sum/3
  Sum/1 -> pb1Filt/1, Delay4/1, Delay/1  "pb1_filt"
  Gain1/1 -> Sum/4
  Delay/1 -> Gain/1
  pb1Meas/1 -> Delay4/2, Delay/2, Delay2/1, Delay2/2, Delay1/1, Delay3/2, Delay3/1, Delay1/2  "pb1Meas"

== system VDCHyd2020a/sbVDCController/sbFormingControlActions/sbpb2LowPassFilter ==
  pb2Meas : Inport
  Delay : Delay  InitialConditionSource=Input port  SampleTime=filtPres.dT
      settings: InputPortMap=u0,p4
  Delay1 : Delay  DelayLength=1  InitialConditionSource=Input port  SampleTime=filtPres.dT
      settings: InputPortMap=u0,p4
  Delay2 : Delay  DelayLength=0  InitialConditionSource=Input port  SampleTime=filtPres.dT
      settings: InputPortMap=u0,p4
  Delay3 : Delay  InitialConditionSource=Input port  SampleTime=filtPres.dT
      settings: InputPortMap=u0,p4
  Delay4 : Delay  DelayLength=1  InitialConditionSource=Input port  SampleTime=filtPres.dT
      settings: InputPortMap=u0,p4
  Gain : Gain  Gain=filtPres.a0
  Gain1 : Gain  Gain=filtPres.b1
  Gain2 : Gain  Gain=filtPres.b2
  Gain3 : Gain  Gain=filtPres.b0
  Gain4 : Gain  Gain=filtPres.a1
  Sum : Sum  Inputs=|--+++
  pb2Filt : Outport
  wires:
  pb2Meas/1 -> Delay4/2, Delay/2, Delay2/1, Delay2/2, Delay1/1, Delay3/2, Delay3/1, Delay1/2  "pb2_meas"
  Sum/1 -> pb2Filt/1, Delay4/1, Delay/1  "pb2_filt"
  Gain2/1 -> Sum/3
  Gain4/1 -> Sum/1
  Delay3/1 -> Gain3/1
  Gain3/1 -> Sum/5
  Delay2/1 -> Gain2/1
  Delay4/1 -> Gain4/1
  Gain/1 -> Sum/2
  Delay/1 -> Gain/1
  Delay1/1 -> Gain1/1
  Gain1/1 -> Sum/4

== system VDCHyd2020a/sbVDCController/sbFormingControlActions/sbpbt2LowPassFilter ==
  pbt2Meas : Inport
  Delay : Delay  InitialConditionSource=Input port  SampleTime=filtPres.dT
      settings: InputPortMap=u0,p4
  Delay1 : Delay  DelayLength=1  InitialConditionSource=Input port  SampleTime=filtPres.dT
      settings: InputPortMap=u0,p4
  Delay2 : Delay  DelayLength=0  InitialConditionSource=Input port  SampleTime=filtPres.dT
      settings: InputPortMap=u0,p4
  Delay3 : Delay  InitialConditionSource=Input port  SampleTime=filtPres.dT
      settings: InputPortMap=u0,p4
  Delay4 : Delay  DelayLength=1  InitialConditionSource=Input port  SampleTime=filtPres.dT
      settings: InputPortMap=u0,p4
  Gain : Gain  Gain=filtPres.a0
  Gain1 : Gain  Gain=filtPres.b1
  Gain2 : Gain  Gain=filtPres.b2
  Gain3 : Gain  Gain=filtPres.b0
  Gain4 : Gain  Gain=filtPres.a1
  Sum : Sum  Inputs=|--+++
  pbt2Filt : Outport
  wires:
  Delay/1 -> Gain/1
  Gain1/1 -> Sum/4
  Sum/1 -> pbt2Filt/1, Delay4/1, Delay/1  "pbt2Filt"
  Gain2/1 -> Sum/3
  Delay4/1 -> Gain4/1
  Delay1/1 -> Gain1/1
  Delay2/1 -> Gain2/1
  Gain/1 -> Sum/2
  pbt2Meas/1 -> Delay4/2, Delay/2, Delay2/1, Delay2/2, Delay1/1, Delay3/2, Delay3/1, Delay1/2  "pbt2Meas"
  Delay3/1 -> Gain3/1
  Gain3/1 -> Sum/5
  Gain4/1 -> Sum/1

== system VDCHyd2020a/sbHydraulicManipulatorSimscape/sbLiftCylinderAndLiftPiston/sbFrictionForceRS1/sbFrictionRegressorRS1 ==
  note: (40) in Zhu, Piedboeuf (2005)
  note: (4) in Zhu, Piedboeuf (2005)
  note: (71) and (72) in Zhu, Piedboeuf (2005)
  dx1 : Inport
  fp1 : Inport  Port=2
  frictionRegressorFunctionRS1 : MATLAB Function  TreatAsAtomicUnit=on
  sbAverageDeformationOfBristlesRS2 : Subsystem
  sbFrictionSwitchingFunctionRS2 : Subsystem
  Yf1 : Outport
  wires:
  dx1/1 -> [dx1]  "dx1"
  [dx1] -> sbAverageDeformationOfBristlesRS2/1(dx1)  "dx1"
  sbAverageDeformationOfBristlesRS2/1(z1) -> [z1]  "z1"
  [dx1] -> sbFrictionSwitchingFunctionRS2/1(dx1)  "dx1"
  sbFrictionSwitchingFunctionRS2/1(LRS1) -> [LRS1]  "LRS1"
  [dx1] -> frictionRegressorFunctionRS1/1(v)  "dx1"
  [z1] -> frictionRegressorFunctionRS1/2(z)  "z1"
  [LRS1] -> frictionRegressorFunctionRS1/3(L)  "LRS1"
  fp1/1 -> [fp1]  "fp1"
  [fp1] -> frictionRegressorFunctionRS1/4(Fd)  "fp1"
  frictionRegressorFunctionRS1/1(Yf) -> [Yf1]  "Yf1"
  [Yf1] -> Yf1/1  "Yf1"

== system VDCHyd2020a/sbHydraulicManipulatorSimscape/sbPrismaticJointCylinderAndPiston/sbFrictionForcePS2/sbFrictionRegressorPS2 ==
  note: (40) in Zhu, Piedboeuf (2005)
  note: (4) in Zhu, Piedboeuf (2005)
  note: (71) and (72) in Zhu, Piedboeuf (2005)
  dxt2 : Inport
  fpt2 : Inport  Port=2
  frictionRegressorFunctionPS2 : MATLAB Function  TreatAsAtomicUnit=on
  sbAverageDeformationOfBristlesPS2 : Subsystem
  sbFrictionSwitchingFunctionPS2 : Subsystem
  Yft2 : Outport
  wires:
  dxt2/1 -> [dxt2]  "dxt2"
  [dxt2] -> sbAverageDeformationOfBristlesPS2/1(dxt2)  "dxt2"
  sbAverageDeformationOfBristlesPS2/1(zt2) -> [zt2]  "zt2"
  [dxt2] -> sbFrictionSwitchingFunctionPS2/1(dxt2)  "dxt2"
  sbFrictionSwitchingFunctionPS2/1(LPS2) -> [LPS2]  "LPS2"
  [dxt2] -> frictionRegressorFunctionPS2/1(v)  "dxt2"
  [zt2] -> frictionRegressorFunctionPS2/2(z)  "zt2"
  [LPS2] -> frictionRegressorFunctionPS2/3(L)  "LPS2"
  fpt2/1 -> [fpt2]  "fpt2"
  [fpt2] -> frictionRegressorFunctionPS2/4(Fd)  "fpt2"
  frictionRegressorFunctionPS2/1(Yf) -> [Yft2]  "Yft2"
  [Yft2] -> Yft2/1  "Yft2"

== system VDCHyd2020a/sbHydraulicManipulatorSimscape/sbTiltCylinderAndTiltPiston/sbFrictionForceRS2/sbFrictionRegressorRS2 ==
  note: (40) in Zhu, Piedboeuf (2005)
  note: (4) in Zhu, Piedboeuf (2005)
  note: (71) and (72) in Zhu, Piedboeuf (2005)
  dx2 : Inport
  fp2 : Inport  Port=2
  frictionRegressorFunctionRS2 : MATLAB Function  TreatAsAtomicUnit=on
  sbAverageDeformationOfBristlesRS2 : Subsystem
  sbFrictionSwitchingFunctionRS2 : Subsystem
  Yf2 : Outport
  wires:
  dx2/1 -> [dx2]  "dx2"
  [dx2] -> sbAverageDeformationOfBristlesRS2/1(dx2)  "dx2"
  sbAverageDeformationOfBristlesRS2/1(z2) -> [z2]  "z2"
  [dx2] -> sbFrictionSwitchingFunctionRS2/1(dx2)  "dx2"
  sbFrictionSwitchingFunctionRS2/1(LRS2) -> [LRS2]  "LRS2"
  [dx2] -> frictionRegressorFunctionRS2/1(v)  "dx2"
  [z2] -> frictionRegressorFunctionRS2/2(z)  "z2"
  [LRS2] -> frictionRegressorFunctionRS2/3(L)  "LRS2"
  fp2/1 -> [fp2]  "fp2"
  [fp2] -> frictionRegressorFunctionRS2/4(Fd)  "fp2"
  frictionRegressorFunctionRS2/1(Yf) -> [Yf2]  "Yf2"
  [Yf2] -> Yf2/1  "Yf2"

== system VDCHyd2020a/sbVDCController/sbFormAnalyticQuantities/sbPrismaticSegment2/sbGeomPropPS2 ==
  note: Get inputs...
  note: Process data...
  note: Pass to outputs...
  xt2 : Inport
  Bus Creator : BusCreator  Inputs=xt2,dxt2
  sbDiscreteDerivative : Subsystem
  geomPropPS2 : Outport
  wires:
  xt2/1 -> [xt2]  "xt2"
  [xt2] -> sbDiscreteDerivative/1(xt2)  "xt2"
  sbDiscreteDerivative/1(xt2Velocity) -> [dxt2]  "dxt2"
  [xt2] -> Bus Creator/1  "xt2"
  [dxt2] -> Bus Creator/2  "dxt2"
  Bus Creator/1 -> [geomPropPS2]  "geomPropPS2"
  [geomPropPS2] -> geomPropPS2/1  "geomPropPS2"

== system VDCHyd2020a/sbVDCController/sbFormAnalyticQuantities/sbPrismaticSegment2/sbPosVecsPS2 ==
  note: Get inputs...
  note: Process data...
  note: Form new buses...
  note: Pass to outputs...
  xt2 : Inport
  Bus Creator : BusCreator  Inputs=P22_r_P22B52,B52_r_B52P32,P32_r_P32D22
  Constant : Constant  Value=posVec.B52_r_B52P32
  Constant1 : Constant  Value=posVec.P32_r_P32D22
  P22_r_P22B52 : MATLAB Function  TreatAsAtomicUnit=on
  posVecsPS2 : Outport
  wires:
  [rP32D22] -> Bus Creator/3  "P32_r_P32D22"
  Constant1/1 -> [rP32D22]  "P32_r_P32D22"
  [PosVecsS2P] -> posVecsPS2/1  "posVecsPS2"
  Bus Creator/1 -> [PosVecsS2P]  "posVecsPS2"
  [rB52P32] -> Bus Creator/2  "B52_r_B52P32"
  [rP22B52] -> Bus Creator/1  "P22_r_P22B52"
  Constant/1 -> [rB52P32]  "B52_r_B52P32"
  P22_r_P22B52/1(P22_r_P22B52) -> [rP22B52]  "P22_r_P22B52"
  [xt2] -> P22_r_P22B52/1(xt2)
  xt2/1 -> [xt2]  "xt2"
